simulink model "CompensationPartielle"  (R2017a)
settings: Solver=VariableStepAuto  StartTime=0.0  StopTime=100  RelTol=1e-3
settings Model: Creator=PC  LastModifiedBy=PC

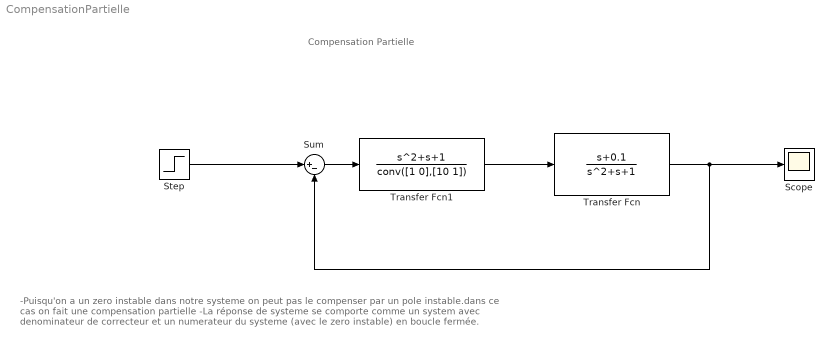
== system CompensationPartielle ==
  note: -Puisqu'on a un zero instable dans notre systeme on peut pas le compenser par un pole instable.dans ce cas on fait une compensation partielle
      | -La réponse de systeme se comporte comme un system avec denominateur de correcteur et un numerateur du systeme (avec le zero instable) en boucle fermée.
  note: Compensation Partielle
  Scope : Scope
  Step : Step  Time=0  SampleTime=0
  Sum : Sum  Inputs=|+-
  Transfer Fcn : TransferFcn  Numerator=[1 0.1]  Denominator=[1 1 1]
  Transfer Fcn1 : TransferFcn  Numerator=[1 1 1]  Denominator=conv([1 0],[10 1])
  wires:
  Step/1 -> Sum/1
  Sum/1 -> Transfer Fcn1/1
  Transfer Fcn/1 -> Sum/2, Scope/1
  Transfer Fcn1/1 -> Transfer Fcn/1
